simulink model "EST_fixed"  (R2025a)
settings: Solver=FixedStepAuto  StartTime=0.0  StopTime=stopt  FixedStep=deltat  MaxStep=0.05  RelTol=1e-3
InitFcn:
  | clear all;
  | close all;
  | clc;
  | 
  | % add the data and script directories
  | addpath('data','scripts');
  | 
  | % load the constants (units)
  | constants;
  | 
  | % load the simulation parameters
  | preprocessing;
StopFcn:
  | postprocessing;
values from neighbouring files (symbols this model uses):
  alphaLoss = 0.1    [preprocessing.m]
  areaTank = 6 * (sideLength^2)    (= 57.9293630763)    [preprocessing.m]
  cableArea = 6e-6    (= 6e-06)    [preprocessing.m]
  cableLength = 28.5    [preprocessing.m]
  cableLengthDemand = 20    [preprocessing.m]
  cableResistivity = 1.676e-8    (= 1.676e-08)    [preprocessing.m]
  cps = 920    [preprocessing.m]
  current = 20    [preprocessing.m]
  currentDemand = 2.5    [preprocessing.m]
  dh_ads = 2.5e6    (= 2500000)    [preprocessing.m]
  E = 6000    [preprocessing.m]
  efficiencyInjection = 0.98    [preprocessing.m]
  emissivitySurface = 0.5    [preprocessing.m]
  emissivitySurfacePipe = 0.9    [preprocessing.m]
  EStorageMax = 2000.*unit("kWh")    [preprocessing.m]
  EStorageMin = 10.*unit("kWh")    [preprocessing.m]
  hAir = 10    [preprocessing.m]
  kInsulation = 0.04    [preprocessing.m]
  kLdf = 0.008    [preprocessing.m]
  kPipe = 0.3    [preprocessing.m]
  kSteel = 54    [preprocessing.m]
  mCpTotal = (massGel * heatCapacityGel) + (massSteel * heatCapacitySteel)    (= 21486379.4261)    [preprocessing.m]
  ms = 20    [preprocessing.m]
  n = 1.5    [preprocessing.m]
  pipeLength = 10    [preprocessing.m]
  pv = 1200    [preprocessing.m]
  r1 = 0.03    [preprocessing.m]
  r2 = 0.035    [preprocessing.m]
  r3 = 0.05    [preprocessing.m]
  stefanBoltz = 5.67e-8    (= 5.67e-08)    [preprocessing.m]
  tempEnv = 293.15    [preprocessing.m]
  Tfluid = 353.15    [preprocessing.m]
  thicknessInsulation = 0.10    (= 0.1)    [preprocessing.m]
  thicknessSteel = 0.015    [preprocessing.m]
  Tref = 373    [preprocessing.m]
  UA = 15    [preprocessing.m]
  X0 = 0.35    [preprocessing.m]
  Xref = 0.75    [preprocessing.m]
settings Model: Creator=joche  LastModifiedBy=20253258
settings DataIOCC: SaveFormat=Array  SaveOutput=off  ReturnWorkspaceOutputs=off
settings OptimizationCC: ReuseModelBlockBuffer=off
settings ModelReferenceCC: EnableRefExpFcnMdlSchedulingChecks=on
settings RTWCC: GPUComputeCapability=3.5

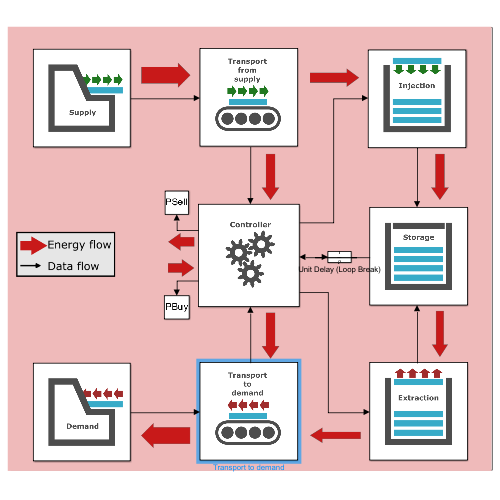
[thumbnail: Simulink's stored preview of the top-level diagram]
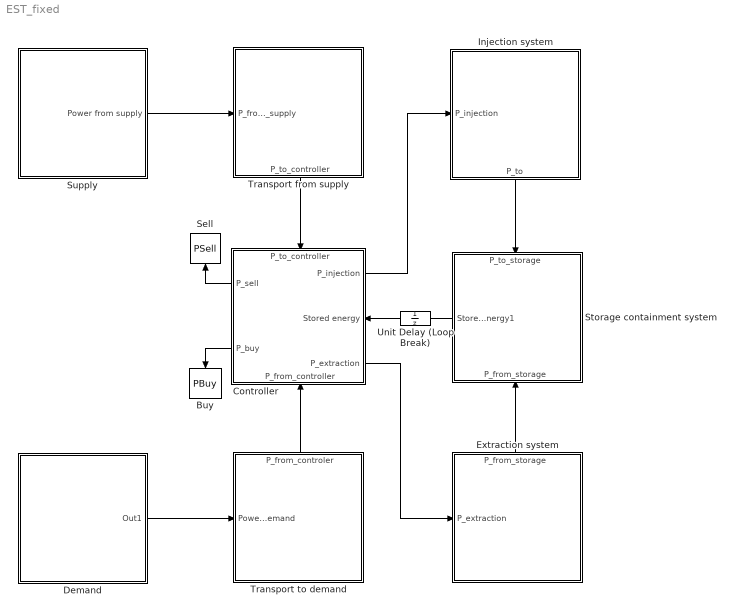
== system EST_fixed ==
  Buy : ToWorkspace  VariableName=PBuy  SampleTime=-1
  Controller : Subsystem
      settings: PortSchema="{\"entries\":[{\"content\":{\"sides\":[{\"content\":{\"connectorIds\":[\"Out3\",\"Out4\"]},\"type\":\"ConnectorPlacement.EquallySpacedRectSide\",\"uuid\":\"4daf33ce-c96a-4783-b5c4-228eed953e01\"},{\"content\":{\"connectorIds\":[\"Out1\",\"In3\",\"Out2\"],\"side\":\"RIGHT\"},\"type\":\"ConnectorPlacement.EquallySpacedRectSide\",\"uuid\":\"e9942e50-8467-4af8-b79b-80636cbc76e5\"},{\"content\":{\"connectorIds\":[\"In1\"],\"side\":\"TOP\"},\"type\":\"ConnectorPlacement.EquallySpacedRectSide\",\"uuid\":\"f315e931-d69b-4751-b712-f89c6c81baeb\"},{\"content\":{\"connectorIds\":[\"In2\"],\"side\":\"BOTTOM\"},\"type\":\"ConnectorPlacement.EquallySpacedRectSide\",\"uuid\":\"44715ee6-5cd5-4669-bcb9-5ed7c869bdb3\"}]},\"type\":\"ConnectorPlacement.EquallySpacedConnector\",\"uuid\":\"fff48899-944b-4064-b7d7-ecc12144fb48\"}],\"packageUris\":[\"http://schema.mathworks.com/mf0/Connector/R2020b\"],\"version\":\"1.0\"}"
      mask Display: image('$imagefile'); % Use "Edit Image" on toolstrip to change.
  Demand : Subsystem
      mask Display: image('$imagefile'); % Use "Edit Image" on toolstrip to change.
  Extraction system : Subsystem
      settings: PortSchema="{\"entries\":[{\"content\":{\"sides\":[{\"content\":{\"connectorIds\":[]},\"type\":\"ConnectorPlacement.EquallySpacedRectSide\",\"uuid\":\"05c5933d-55fc-4e06-853f-fc26d42905f9\"},{\"content\":{\"connectorIds\":[\"In1\"],\"side\":\"RIGHT\"},\"type\":\"ConnectorPlacement.EquallySpacedRectSide\",\"uuid\":\"327426c5-31d5-498b-a2bd-83e49353408c\"},{\"content\":{\"connectorIds\":[],\"side\":\"TOP\"},\"type\":\"ConnectorPlacement.EquallySpacedRectSide\",\"uuid\":\"55306cf3-a3de-4385-a5ae-b8600ecdd5a2\"},{\"content\":{\"connectorIds\":[\"Out1\"],\"side\":\"BOTTOM\"},\"type\":\"ConnectorPlacement.EquallySpacedRectSide\",\"uuid\":\"08fcc9c3-40d3-4ac6-b914-dfeef6039ffb\"}]},\"type\":\"ConnectorPlacement.EquallySpacedConnector\",\"uuid\":\"cb35d5ba-e8c6-462c-b7b2-fe8356d4b0a1\"}],\"packageUris\":[\"http://schema.mathworks.com/mf0/Connector/R2020b\"],\"version\":\"1.0\"}"
      mask Display: image('$imagefile'); % Use "Edit Image" on toolstrip to change.
  Injection system : Subsystem
      settings: PortSchema="{\"entries\":[{\"content\":{\"sides\":[{\"content\":{\"connectorIds\":[]},\"type\":\"ConnectorPlacement.EquallySpacedRectSide\",\"uuid\":\"05c5933d-55fc-4e06-853f-fc26d42905f9\"},{\"content\":{\"connectorIds\":[\"In1\"],\"side\":\"RIGHT\"},\"type\":\"ConnectorPlacement.EquallySpacedRectSide\",\"uuid\":\"327426c5-31d5-498b-a2bd-83e49353408c\"},{\"content\":{\"connectorIds\":[\"Out1\"],\"side\":\"TOP\"},\"type\":\"ConnectorPlacement.EquallySpacedRectSide\",\"uuid\":\"55306cf3-a3de-4385-a5ae-b8600ecdd5a2\"},{\"content\":{\"connectorIds\":[],\"side\":\"BOTTOM\"},\"type\":\"ConnectorPlacement.EquallySpacedRectSide\",\"uuid\":\"08fcc9c3-40d3-4ac6-b914-dfeef6039ffb\"}]},\"type\":\"ConnectorPlacement.EquallySpacedConnector\",\"uuid\":\"cb35d5ba-e8c6-462c-b7b2-fe8356d4b0a1\"}],\"packageUris\":[\"http://schema.mathworks.com/mf0/Connector/R2020b\"],\"version\":\"1.0\"}"
      mask Display: image('$imagefile'); % Use "Edit Image" on toolstrip to change.
  Sell : ToWorkspace  VariableName=PSell  SampleTime=-1
  Storage containment system : Subsystem
      settings: PortSchema="{\"entries\":[{\"content\":{\"sides\":[{\"content\":{\"connectorIds\":[\"Out1\"]},\"type\":\"ConnectorPlacement.EquallySpacedRectSide\",\"uuid\":\"0ba48424-33b9-4934-970f-64fe5d8b070e\"},{\"content\":{\"connectorIds\":[],\"side\":\"RIGHT\"},\"type\":\"ConnectorPlacement.EquallySpacedRectSide\",\"uuid\":\"9cde340f-8f39-4499-9a12-5e1623737660\"},{\"content\":{\"connectorIds\":[\"In1\"],\"side\":\"TOP\"},\"type\":\"ConnectorPlacement.EquallySpacedRectSide\",\"uuid\":\"2af8db04-7fd0-4902-8637-8dc00edb4598\"},{\"content\":{\"connectorIds\":[\"In2\"],\"side\":\"BOTTOM\"},\"type\":\"ConnectorPlacement.EquallySpacedRectSide\",\"uuid\":\"e21ea806-d777-41a3-a53f-556fae66854b\"}]},\"type\":\"ConnectorPlacement.EquallySpacedConnector\",\"uuid\":\"4e2ddb36-4db3-4ab4-858b-ebb8ccefeb1f\"}],\"packageUris\":[\"http://schema.mathworks.com/mf0/Connector/R2020b\"],\"version\":\"1.0\"}"
      mask Display: image('$imagefile'); % Use "Edit Image" on toolstrip to change.
  Supply : Subsystem
      mask Display: image('$imagefile'); % Use "Edit Image" on toolstrip to change.
  Transport from supply : Subsystem
      settings: PortSchema="{\"entries\":[{\"content\":{\"sides\":[{\"content\":{\"connectorIds\":[\"In1\"]},\"type\":\"ConnectorPlacement.EquallySpacedRectSide\",\"uuid\":\"31329006-3d36-4d93-9c44-7503a515d397\"},{\"content\":{\"connectorIds\":[],\"side\":\"RIGHT\"},\"type\":\"ConnectorPlacement.EquallySpacedRectSide\",\"uuid\":\"aba139c7-f9b6-4881-a56b-a4cbbedacd88\"},{\"content\":{\"connectorIds\":[],\"side\":\"TOP\"},\"type\":\"ConnectorPlacement.EquallySpacedRectSide\",\"uuid\":\"e683eb73-7a35-4160-9c39-da83856a6278\"},{\"content\":{\"connectorIds\":[\"Out1\"],\"side\":\"BOTTOM\"},\"type\":\"ConnectorPlacement.EquallySpacedRectSide\",\"uuid\":\"1170dd18-447c-437f-9043-6812c2877331\"}]},\"type\":\"ConnectorPlacement.EquallySpacedConnector\",\"uuid\":\"804af608-1d70-444f-af69-e05f19bf98f3\"}],\"packageUris\":[\"http://schema.mathworks.com/mf0/Connector/R2020b\"],\"version\":\"1.0\"}"
      mask Display: image('$imagefile'); % Use "Edit Image" on toolstrip to change.
  Transport to demand : Subsystem
      settings: PortSchema="{\"entries\":[{\"content\":{\"sides\":[{\"content\":{\"connectorIds\":[\"In1\"]},\"type\":\"ConnectorPlacement.EquallySpacedRectSide\",\"uuid\":\"31329006-3d36-4d93-9c44-7503a515d397\"},{\"content\":{\"connectorIds\":[],\"side\":\"RIGHT\"},\"type\":\"ConnectorPlacement.EquallySpacedRectSide\",\"uuid\":\"aba139c7-f9b6-4881-a56b-a4cbbedacd88\"},{\"content\":{\"connectorIds\":[\"Out1\"],\"side\":\"TOP\"},\"type\":\"ConnectorPlacement.EquallySpacedRectSide\",\"uuid\":\"e683eb73-7a35-4160-9c39-da83856a6278\"},{\"content\":{\"connectorIds\":[],\"side\":\"BOTTOM\"},\"type\":\"ConnectorPlacement.EquallySpacedRectSide\",\"uuid\":\"c378138f-7233-4483-870c-40a69b3495ee\"}]},\"type\":\"ConnectorPlacement.EquallySpacedConnector\",\"uuid\":\"804af608-1d70-444f-af69-e05f19bf98f3\"}],\"packageUris\":[\"http://schema.mathworks.com/mf0/Connector/R2020b\"],\"version\":\"1.0\"}"
      mask Display: image('$imagefile'); % Use "Edit Image" on toolstrip to change.
  Unit Delay (Loop Break) : UnitDelay  SampleTime=-1
  wires:
  Supply/1(Power from supply) -> Transport from supply/1(P_from_supply)
  Transport from supply/1(P_to_controller) -> Controller/1(P_to_controller)
  Transport to demand/1(P_from_controler) -> Controller/2(P_from_controller)
  Demand/1(Out1) -> Transport to demand/1(Power to demand)
  Controller/3(P_sell) -> Sell/1
  Controller/2(P_extraction) -> Extraction system/1(P_extraction)
  Injection system/1(P_to) -> Storage containment system/1(P_to_storage)
  Extraction system/1(P_from_storage) -> Storage containment system/2(P_from_storage)
  Storage containment system/1(Stored energy1) -> Unit Delay (Loop Break)/1
  Unit Delay (Loop Break)/1 -> Controller/3(Stored energy)
  Controller/1(P_injection) -> Injection system/1(P_injection)
  Controller/4(P_buy) -> Buy/1

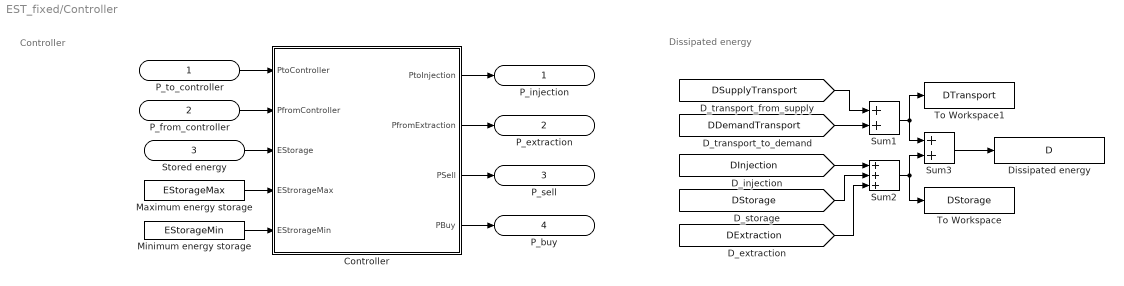
== system EST_fixed/Controller ==
  note: Dissipated energy
  note: Controller
  P_to_controller : Inport
  P_from_controller : Inport  Port=2
  Stored energy : Inport  Port=3
  Controller : MATLAB Function  TreatAsAtomicUnit=on
  Dissipated energy : ToWorkspace  VariableName=D  SampleTime=-1
  Maximum energy storage : Constant  Value=EStorageMax
  Minimum energy storage : Constant  Value=EStorageMin
  Sum1 : Sum
  Sum2 : Sum  Inputs=+++
  Sum3 : Sum
  To Workspace : ToWorkspace  VariableName=DStorage  SampleTime=-1
  To Workspace1 : ToWorkspace  VariableName=DTransport  SampleTime=-1
  P_injection : Outport
  P_extraction : Outport  Port=2
  P_sell : Outport  Port=3
  P_buy : Outport  Port=4
  wires:
  P_from_controller/1 -> Controller/2(PfromController)
  Controller/2(PfromExtraction) -> P_extraction/1
  Controller/3(PSell) -> P_sell/1
  Controller/4(PBuy) -> P_buy/1
  Minimum energy storage/1 -> Controller/5(EStrorageMin)
  Maximum energy storage/1 -> Controller/4(EStrorageMax)
  P_to_controller/1 -> Controller/1(PtoController)
  Controller/1(PtoInjection) -> P_injection/1
  Stored energy/1 -> Controller/3(EStorage)
  [DDemandTransport] -> Sum1/2
  [DSupplyTransport] -> Sum1/1
  [DInjection] -> Sum2/1
  [DStorage] -> Sum2/2
  [DExtraction] -> Sum2/3
  Sum2/1 -> To Workspace/1, Sum3/2
  Sum1/1 -> To Workspace1/1, Sum3/1
  Sum3/1 -> Dissipated energy/1

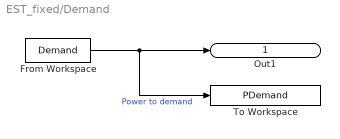
== system EST_fixed/Demand ==
  From Workspace : FromWorkspace  VariableName=Demand  OutputAfterFinalValue=Setting to zero
  To Workspace : ToWorkspace  VariableName=PDemand  SampleTime=-1
  Out1 : Outport
  wires:
  From Workspace/1 -> To Workspace/1, Out1/1  "Power to demand"

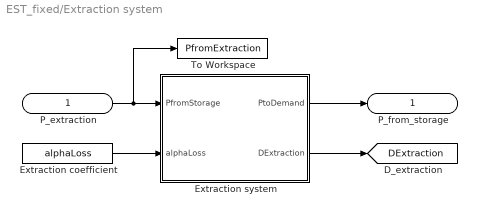
== system EST_fixed/Extraction system ==
  P_extraction : Inport
  Extraction coefficient : Constant  Value=alphaLoss
  Extraction system : MATLAB Function  TreatAsAtomicUnit=on
  To Workspace : ToWorkspace  VariableName=PfromExtraction  SampleTime=-1
  P_from_storage : Outport
  tag scope: DExtraction=global
  wires:
  P_extraction/1 -> To Workspace/1, Extraction system/1(PfromStorage)
  Extraction system/1(PtoDemand) -> P_from_storage/1
  Extraction system/2(DExtraction) -> [DExtraction]
  Extraction coefficient/1 -> Extraction system/2(alphaLoss)

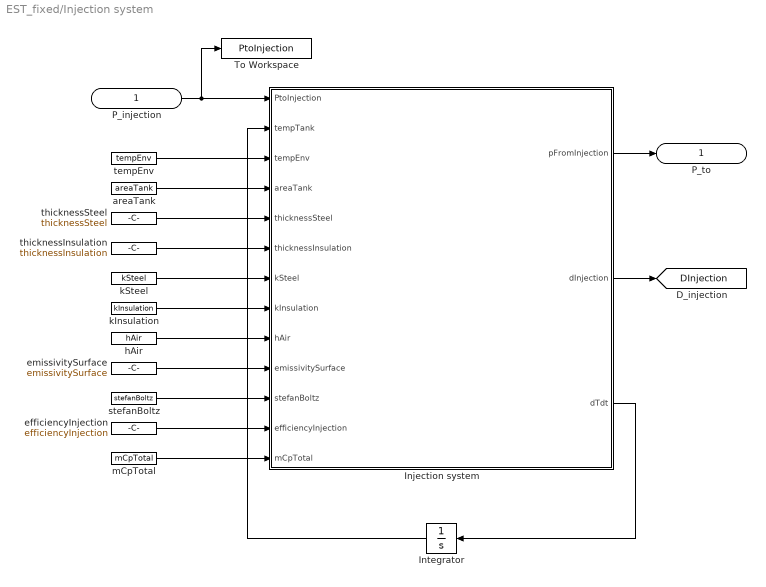
== system EST_fixed/Injection system ==
  P_injection : Inport
  Injection system : MATLAB Function  TreatAsAtomicUnit=on
  Integrator : Integrator  InitialCondition=293.15
  To Workspace : ToWorkspace  VariableName=PtoInjection  SampleTime=-1
  areaTank : Constant  Value=areaTank
  efficiencyInjection : Constant  Value=efficiencyInjection
  emissivitySurface : Constant  Value=emissivitySurface
  hAir : Constant  Value=hAir
  kInsulation : Constant  Value=kInsulation
  kSteel : Constant  Value=kSteel
  mCpTotal : Constant  Value=mCpTotal
  stefanBoltz : Constant  Value=stefanBoltz
  tempEnv : Constant  Value=tempEnv
  thicknessInsulation : Constant  Value=thicknessInsulation
  thicknessSteel : Constant  Value=thicknessSteel
  P_to : Outport
  tag scope: DInjection=global
  wires:
  P_injection/1 -> Injection system/1(PtoInjection), To Workspace/1
  Injection system/1(pFromInjection) -> P_to/1
  Injection system/2(dInjection) -> [DInjection]
  Injection system/3(dTdt) -> Integrator/1
  Integrator/1 -> Injection system/2(tempTank)
  tempEnv/1 -> Injection system/3(tempEnv)
  areaTank/1 -> Injection system/4(areaTank)
  thicknessSteel/1 -> Injection system/5(thicknessSteel)
  thicknessInsulation/1 -> Injection system/6(thicknessInsulation)
  kSteel/1 -> Injection system/7(kSteel)
  kInsulation/1 -> Injection system/8(kInsulation)
  hAir/1 -> Injection system/9(hAir)
  emissivitySurface/1 -> Injection system/10(emissivitySurface)
  stefanBoltz/1 -> Injection system/11(stefanBoltz)
  efficiencyInjection/1 -> Injection system/12(efficiencyInjection)
  mCpTotal/1 -> Injection system/13(mCpTotal)

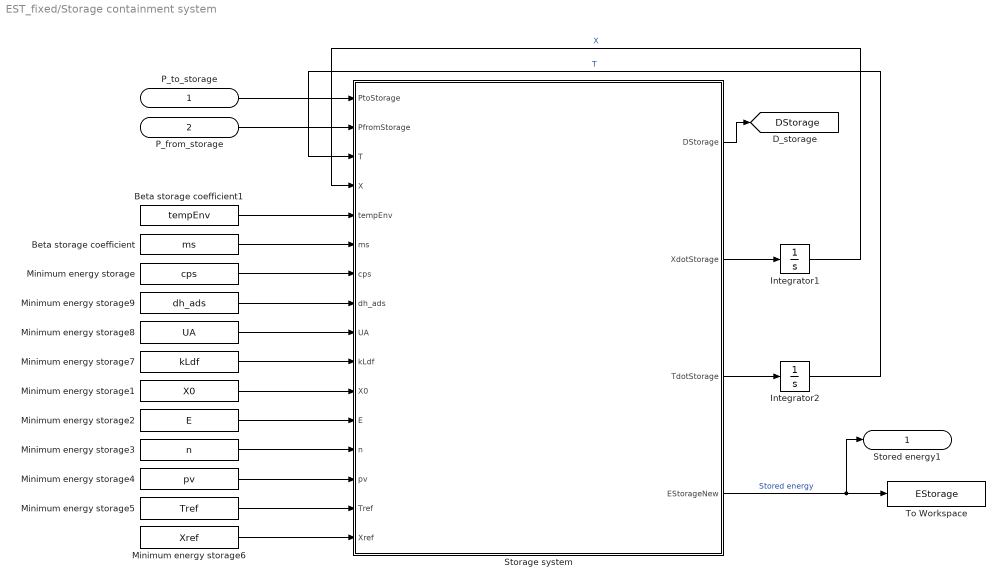
== system EST_fixed/Storage containment system ==
  P_to_storage : Inport
  P_from_storage : Inport  Port=2
  Beta storage coefficient : Constant  Value=ms
  Beta storage coefficient1 : Constant  Value=tempEnv
  Integrator1 : Integrator  InitialCondition=0.05
  Integrator2 : Integrator  InitialCondition=tempEnv
  Minimum energy storage : Constant  Value=cps
  Minimum energy storage1 : Constant  Value=X0
  Minimum energy storage2 : Constant  Value=E
  Minimum energy storage3 : Constant  Value=n
  Minimum energy storage4 : Constant  Value=pv
  Minimum energy storage5 : Constant  Value=Tref
  Minimum energy storage6 : Constant  Value=Xref
  Minimum energy storage7 : Constant  Value=kLdf
  Minimum energy storage8 : Constant  Value=UA
  Minimum energy storage9 : Constant  Value=dh_ads
  Storage system : MATLAB Function  TreatAsAtomicUnit=on
  To Workspace : ToWorkspace  VariableName=EStorage  SampleTime=-1
  Stored energy1 : Outport
  tag scope: DStorage=global
  wires:
  P_from_storage/1 -> Storage system/2(PfromStorage)
  P_to_storage/1 -> Storage system/1(PtoStorage)
  Storage system/4(EStorageNew) -> Stored energy1/1, To Workspace/1  "Stored energy"
  Storage system/1(DStorage) -> [DStorage]
  Beta storage coefficient/1 -> Storage system/6(ms)
  Minimum energy storage/1 -> Storage system/7(cps)
  Minimum energy storage1/1 -> Storage system/11(X0)
  Minimum energy storage2/1 -> Storage system/12(E)
  Minimum energy storage3/1 -> Storage system/13(n)
  Minimum energy storage4/1 -> Storage system/14(pv)
  Minimum energy storage7/1 -> Storage system/10(kLdf)
  Minimum energy storage8/1 -> Storage system/9(UA)
  Beta storage coefficient1/1 -> Storage system/5(tempEnv)
  Minimum energy storage9/1 -> Storage system/8(dh_ads)
  Storage system/2(XdotStorage) -> Integrator1/1
  Integrator1/1 -> Storage system/4(X)  "X"
  Storage system/3(TdotStorage) -> Integrator2/1
  Integrator2/1 -> Storage system/3(T)  "T"
  Minimum energy storage5/1 -> Storage system/15(Tref)
  Minimum energy storage6/1 -> Storage system/16(Xref)

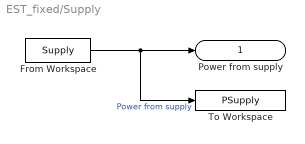
== system EST_fixed/Supply ==
  From Workspace : FromWorkspace  VariableName=Supply  OutputAfterFinalValue=Setting to zero
  To Workspace : ToWorkspace  VariableName=PSupply  SampleTime=-1
  Power from supply : Outport
  wires:
  From Workspace/1 -> To Workspace/1, Power from supply/1  "Power from supply"

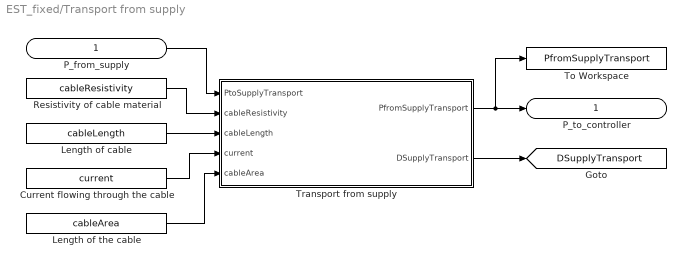
== system EST_fixed/Transport from supply ==
  P_from_supply : Inport
  Current flowing through the cable : Constant  Value=current
  Length of cable : Constant  Value=cableLength
  Length of the cable : Constant  Value=cableArea
  Resistivity of cable material : Constant  Value=cableResistivity
  To Workspace : ToWorkspace  VariableName=PfromSupplyTransport  SampleTime=-1
  Transport from supply : MATLAB Function  TreatAsAtomicUnit=on
  P_to_controller : Outport
  tag scope: DSupplyTransport=global
  wires:
  Transport from supply/1(PfromSupplyTransport) -> To Workspace/1, P_to_controller/1
  Transport from supply/2(DSupplyTransport) -> [DSupplyTransport]
  P_from_supply/1 -> Transport from supply/1(PtoSupplyTransport)
  Resistivity of cable material/1 -> Transport from supply/2(cableResistivity)
  Current flowing through the cable/1 -> Transport from supply/4(current)
  Length of the cable/1 -> Transport from supply/5(cableArea)
  Length of cable/1 -> Transport from supply/3(cableLength)

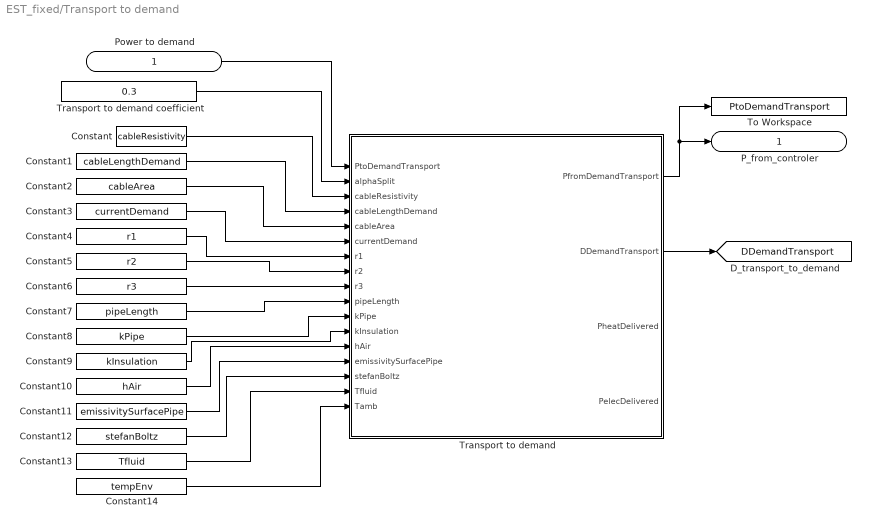
== system EST_fixed/Transport to demand ==
  Power to demand : Inport
  Constant : Constant  Value=cableResistivity
  Constant1 : Constant  Value=cableLengthDemand
  Constant10 : Constant  Value=hAir
  Constant11 : Constant  Value=emissivitySurfacePipe
  Constant12 : Constant  Value=stefanBoltz
  Constant13 : Constant  Value=Tfluid
  Constant14 : Constant  Value=tempEnv
  Constant2 : Constant  Value=cableArea
  Constant3 : Constant  Value=currentDemand
  Constant4 : Constant  Value=r1
  Constant5 : Constant  Value=r2
  Constant6 : Constant  Value=r3
  Constant7 : Constant  Value=pipeLength
  Constant8 : Constant  Value=kPipe
  Constant9 : Constant  Value=kInsulation
  To Workspace : ToWorkspace  VariableName=PtoDemandTransport  SampleTime=-1
  Transport to demand : MATLAB Function  TreatAsAtomicUnit=on
  Transport to demand coefficient : Constant  Value=0.3
  P_from_controler : Outport
  tag scope: DDemandTransport=global
  wires:
  Transport to demand coefficient/1 -> Transport to demand/2(alphaSplit)
  Power to demand/1 -> Transport to demand/1(PtoDemandTransport)
  Transport to demand/1(PfromDemandTransport) -> To Workspace/1, P_from_controler/1
  Transport to demand/2(DDemandTransport) -> [DDemandTransport]
  Constant/1 -> Transport to demand/3(cableResistivity)
  Constant1/1 -> Transport to demand/4(cableLengthDemand)
  Constant2/1 -> Transport to demand/5(cableArea)
  Constant3/1 -> Transport to demand/6(currentDemand)
  Constant4/1 -> Transport to demand/7(r1)
  Constant5/1 -> Transport to demand/8(r2)
  Constant6/1 -> Transport to demand/9(r3)
  Constant7/1 -> Transport to demand/10(pipeLength)
  Constant8/1 -> Transport to demand/11(kPipe)
  Constant9/1 -> Transport to demand/12(kInsulation)
  Constant10/1 -> Transport to demand/13(hAir)
  Constant11/1 -> Transport to demand/14(emissivitySurfacePipe)
  Constant12/1 -> Transport to demand/15(stefanBoltz)
  Constant13/1 -> Transport to demand/16(Tfluid)
  Constant14/1 -> Transport to demand/17(Tamb)

== matlab function EST_fixed/Transport to demand/Transport to demand ==
  data: PtoDemandTransport input; PfromDemandTransport output; alphaSplit input; DDemandTransport output; cableResistivity input; cableLengthDemand input; cableArea input; currentDemand input; r1 input; r2 input; r3 input; pipeLength input; kPipe input; kInsulation input; hAir input; emissivitySurfacePipe input; stefanBoltz input; Tfluid input; Tamb input; PheatDelivered output; PelecDelivered output
function [PfromDemandTransport, DDemandTransport, PheatDelivered, PelecDelivered] = demandTransport( PtoDemandTransport, alphaSplit, cableResistivity, cableLengthDemand, cableArea, currentDemand, r1, r2, r3, pipeLength, kPipe, kInsulation, hAir, emissivitySurfacePipe, stefanBoltz, Tfluid, Tamb)

epsilon = 1e-9;

% ELECTRICAL TRANSPORT 
cableArea_safe = max(cableArea, epsilon);
R = cableResistivity * (2.0 * cableLengthDemand / cableArea_safe);
PlossElec = (currentDemand^2 * R) / 1000.0; % [kW]

alphaSplit_safe = max(0.0, min(1.0, alphaSplit));
Pheat = alphaSplit_safe * PtoDemandTransport;
Pelec = (1.0 - alphaSplit_safe) * PtoDemandTransport;
PelecDelivered = max(0.0, Pelec - PlossElec);

% THERMAL TRANSPORT 
% Clamp temperatures to positive values
Tfluid_safe = max(Tfluid, 1.0);
Tamb_safe   = max(Tamb,   1.0);

% Guard pipe radii ordering: r1 less than r2 less than r3
r1_safe = max(r1, epsilon);
r2_safe = max(r2, 2.0 * r1_safe);
r3_safe = max(r3, 2.0 * r2_safe);

kPipe_safe       = max(kPipe,       epsilon);
kInsulation_safe = max(kInsulation, epsilon);
pipeLength_safe  = max(pipeLength,  epsilon);

% Conduction resistance [K/W]
Rcond = log(r2_safe / r1_safe) / (2.0 * pi * kPipe_safe * pipeLength_safe) ...
      + log(r3_safe / r2_safe) / (2.0 * pi * kInsulation_safe * pipeLength_safe);

% Convection resistance [K/W]
hAir_safe = max(hAir, epsilon);
Aext      = 2.0 * pi * r3_safe * pipeLength_safe;
Rconv     = 1.0 / (hAir_safe * Aext);

% Radiation resistance [K/W]
emiss_safe  = max(emissivitySurfacePipe, epsilon);
stefan_safe = max(stefanBoltz,           epsilon);
Tsum2 = Tfluid_safe^2 + Tamb_safe^2;   % > 0 since temps >= 1K
Tsum1 = Tfluid_safe   + Tamb_safe;      % > 0
Rrad  = 1.0 / (emiss_safe * stefan_safe * Aext * Tsum2 * Tsum1);

% Parallel surface resistance
Rsurf_inv = (1.0 / Rconv) + (1.0 / Rrad);
Rsurf     = 1.0 / max(Rsurf_inv, epsilon);

% Total resistance and heat loss
Rtot         = max(Rcond + Rsurf, epsilon);
PlossHeat_W  = (Tfluid_safe - Tamb_safe) / Rtot;
PlossHeat_kW = PlossHeat_W / 1000.0;

PheatDelivered = max(0.0, Pheat - PlossHeat_kW);

% TOTALS 
DDemandTransport     = PlossElec + PlossHeat_kW;
PfromDemandTransport = PtoDemandTransport - DDemandTransport;

end

== matlab function EST_fixed/Injection system/Injection system ==
  data: PtoInjection input; pFromInjection output; tempTank input; dInjection output; tempEnv input; dTdt output; areaTank input; thicknessSteel input; thicknessInsulation input; kSteel input; kInsulation input; hAir input; emissivitySurface input; stefanBoltz input; efficiencyInjection input; mCpTotal input
function [pFromInjection, dInjection, dTdt] = injection(PtoInjection, tempTank, tempEnv, areaTank, thicknessSteel, thicknessInsulation, kSteel, kInsulation, hAir, emissivitySurface, stefanBoltz, efficiencyInjection, mCpTotal)

epsilon = 1e-9;

% Convert input power from kW to W
PtoInjectionW = PtoInjection * 1000.0;

% Clamp efficiency to [0,1]
efficiencyInjection_safe = max(0.0, min(1.0, efficiencyInjection));
lossConversion = PtoInjectionW * (1.0 - efficiencyInjection_safe);

% Clamp temperatures: must be physically positive
tempTank_safe = max(tempTank, 1.0);
tempEnv_safe  = max(tempEnv,  1.0);

% Guard material and geometry parameters
kSteel_safe      = max(kSteel,      epsilon);
kInsulation_safe = max(kInsulation, epsilon);
areaTank_safe    = max(areaTank,    epsilon);

% Conduction resistance [K/W]
Rcond = (thicknessSteel      / (kSteel_safe      * areaTank_safe)) ...
      + (thicknessInsulation  / (kInsulation_safe * areaTank_safe));

% Convection resistance [K/W]
hAir_safe = max(hAir, epsilon);
Rconv     = 1.0 / (hAir_safe * areaTank_safe);

% Radiation resistance [K/W] - guard temperature product
emiss_safe  = max(emissivitySurface, epsilon);
stefan_safe = max(stefanBoltz,       epsilon);
Tsum2 = tempTank_safe^2 + tempEnv_safe^2;  % > 0 (temps >= 1K)
Tsum1 = tempTank_safe   + tempEnv_safe;     % > 0
Rrad  = 1.0 / (emiss_safe * stefan_safe * areaTank_safe * Tsum2 * Tsum1);

% Parallel surface resistance
Rsurf_inv = (1.0 / Rconv) + (1.0 / Rrad);
Rsurf     = 1.0 / max(Rsurf_inv, epsilon);

% Total resistance and heat loss [W]
Rtot             = max(Rcond + Rsurf, epsilon);
lossHeatTransfer = (tempTank_safe - tempEnv_safe) / Rtot;

% Power balance [W]
dInjectionW     = lossHeatTransfer + lossConversion;
pFromInjectionW = max(0.0, PtoInjectionW - dInjectionW);

% Temperature rate of tank [K/s]
mCpTotal_safe = max(mCpTotal, epsilon);
dTdt_raw = pFromInjectionW / mCpTotal_safe;
dTdt     = max(-100.0, min(100.0, dTdt_raw)); % [K/s] clamp

% Convert back to kW
dInjection     = dInjectionW     / 1000.0;
pFromInjection = pFromInjectionW / 1000.0;

end

== matlab function EST_fixed/Transport from supply/Transport from supply ==
  data: PfromSupplyTransport output; DSupplyTransport output; PtoSupplyTransport input; cableResistivity input; cableLength input; current input; cableArea input
function [PfromSupplyTransport, DSupplyTransport] = supplyTransport(PtoSupplyTransport, cableResistivity, cableLength, current, cableArea)

epsilon = 1e-9;
cableArea_safe = max(cableArea, epsilon);

R = cableResistivity * (2.0 * cableLength / cableArea_safe); % [Ohm]

DSupplyTransport = (current^2 * R) / 1000.0; % [kW]

PfromSupplyTransport = max(0.0, PtoSupplyTransport - DSupplyTransport);

end

== matlab function EST_fixed/Controller/Controller ==
  data: PtoInjection output; PfromExtraction output; PSell output; PBuy output; PtoController input; PfromController input; EStorage input; EStrorageMax input; EStrorageMin input
function [PtoInjection, PfromExtraction, PSell, PBuy] = controller(PtoController, PfromController, EStorage, EStrorageMax, EStrorageMin)
    
    %% Power surplus or deficit

    deltaP = PtoController - PfromController;

    % Power surplus
    if deltaP >= 0

        %% Storage injection

        % Storage system is not full
        if EStorage < EStrorageMax 

            PtoInjection = deltaP;

        % Storage system is full
        else
            PtoInjection = 0;
        end

        %% Storage extraction

        PfromExtraction = 0;

        %% Load-balancing
        PSell   = deltaP - PtoInjection;
        PBuy    = 0;

    % Power deficit
    else

        %% Storage injection

        PtoInjection = 0;

        %% Storage extraction

        % Storage system is not empty
        if EStorage > EStrorageMin

            PfromExtraction = -deltaP;

        % Storage system is empty
        else
            PfromExtraction = 0;
        end

        %% Load-balancing

        PSell = 0;
        PBuy  = -deltaP - PfromExtraction;
    end
end

== matlab function EST_fixed/Extraction system/Extraction system ==
  data: PfromStorage input; PtoDemand output; DExtraction output; alphaLoss input
function [PtoDemand, DExtraction] = extraction(PfromStorage, alphaLoss)

% ORC EFFICIENCY

% etaCarnot = max(0, 1 - Tcond / T);

% etaORC = etaMech * etaCarnot;
% ELECTRICITY OUTPUT

% PtoDemandElec = etaORC * PfromStorage;

% EXTRACTION LOSSES

DExtraction = alphaLoss * PfromStorage;

% HEATING OUTPUT

PtoDemand = PfromStorage - DExtraction;

end

== matlab function EST_fixed/Storage containment system/Storage system ==
  data: DStorage output; PtoStorage input; PfromStorage input; T input; X input; tempEnv input; ms input; cps input; dh_ads input; UA input; XdotStorage output; TdotStorage output; kLdf input; X0 input; E input; n input; pv input; Tref input; Xref input; EStorageNew output
function [DStorage, XdotStorage, TdotStorage, EStorageNew] = Storage( PtoStorage, PfromStorage, T, X, tempEnv, ms, cps, dh_ads, UA, kLdf, X0, E, n, pv, Tref, Xref)

% Universal gas constant
R = 8.314; % [J/(mol*K)]

% Small positive floor used throughout to prevent division by zero
epsilon = 1e-9;

% CLAMPING
T_safe  = max(T,   273.0);          % min 273 K (0 deg C)
X0_safe = max(X0,  epsilon);
X_safe  = max(0.0, min(X0_safe, X)); % loading in [0, X0]

% ---- SATURATION PRESSURE (ANTOINE EQUATION FOR WATER) ----
T_C = T_safe - 273.15;              % Kelvin to Celsius
A   = 8.07131;
B   = 1730.63;
C_antoine = 233.426;

% Guard denominator: singularity when T_C = -C_antoine (~40 K, unphysical)
C_denom = C_antoine + T_C;
if ~(abs(C_denom) > 1e-4)
    C_denom = 1e-4;
end

Psat_mmHg = 10^(A - B / C_denom);  % [mmHg]
psat      = max(Psat_mmHg * 133.322, epsilon); % [Pa]
pv_safe   = max(pv, epsilon);       % [Pa]

% DUBININ-ASTAKHOV EQUILIBRIUM
ratio   = max(psat / pv_safe, 1.0 + epsilon); % always > 1 so log > 0
E_safe  = max(E, epsilon);
n_safe  = max(n, epsilon);          % exponent must be positive

da_arg  = (R * T_safe / E_safe) * log(ratio);
da_base = max(0.0, da_arg);

% Guard exp argument: exp(-500) ~ 0, safe; prevents NaN from -Inf
da_exp_arg = -(da_base ^ n_safe);
da_exp_arg = max(-500.0, da_exp_arg);

Xeq = X0_safe * exp(da_exp_arg);
Xeq = max(0.0, min(X0_safe, Xeq));

%  LINEAR DRIVING FORCE (LDF) KINETICS
kLdf_safe       = max(kLdf, 0.0);
XdotStorage_raw = kLdf_safe * (Xeq - X_safe);
XdotStorage     = max(-10.0, min(10.0, XdotStorage_raw)); % [kg/kg/s] clamp

% HEAT TERMS 
ms_safe   = max(ms,  epsilon);
cps_safe  = max(cps, epsilon);
Qreaction = -ms_safe * dh_ads * XdotStorage;  % [W]
Qloss     = UA * (T_safe - tempEnv);            % [W]

% TEMPERATURE DERIVATIVE 
thermal_mass    = ms_safe * cps_safe;           % [J/K]
Tdot_num        = PtoStorage - PfromStorage + Qreaction - Qloss;
TdotStorage_raw = Tdot_num / thermal_mass;
TdotStorage     = max(-500.0, min(500.0, TdotStorage_raw)); % [K/s] clamp

% STORED ENERGY 
Echemical   = -ms_safe * dh_ads * (X_safe - Xref);
Ethermal    = thermal_mass * (T_safe - Tref);
EStorageNew = Echemical + Ethermal;

% -DISSIPATION
DStorage = Qloss;

end
